simulink model "chap4_5sim"  (Simulink 7.7)
settings: Solver=ode45  StartTime=0.0  StopTime=10  RelTol=1e-5
settings Model: Creator=hp  LastModifiedBy=ljk  ExtModeTrigMode=oneshot  ExtModeArmWhenConnect=off
settings DataIOCC: LimitDataPoints=off  SignalLoggingName=sigsOut
settings OptimizationCC: BooleanDataType=off  InitFltsAndDblsToZero=on
settings DebuggingCC: SaveWithParameterizedLinksMsg=none  SignalResolutionControl=TryResolveAllWithWarning  SolverPrmCheckMsg=none  MultiTaskDSMMsg=warning  MultiTaskCondExecSysMsg=none  StrictBusMsg=None
settings HardwareCC: TargetUnknown=on
settings RTWCC: IncludeERTFirstTime=on
settings GRTTargetCC: TargetFcnLib=ansi_tfl_tmw.mat

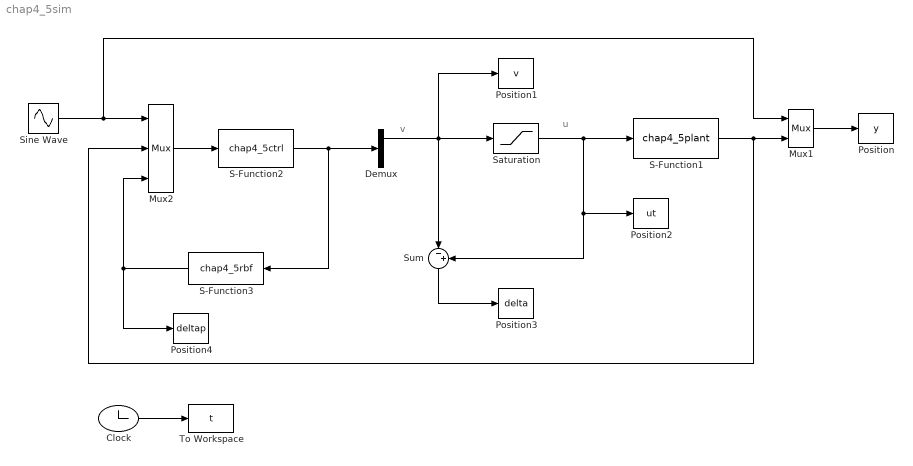
== system chap4_5sim ==
  note: v
  note: u
  Clock : Clock
      settings: Decimation=10
  Demux : Demux  Outputs=2
  Mux1 : Mux  Inputs=2
  Mux2 : Mux  Inputs=3
  Position : ToWorkspace  VariableName=y  SampleTime=-1  SaveFormat=Array
  Position1 : ToWorkspace  VariableName=v  SampleTime=-1  SaveFormat=Array
  Position2 : ToWorkspace  VariableName=ut  SampleTime=-1  SaveFormat=Array
  Position3 : ToWorkspace  VariableName=delta  SampleTime=-1  SaveFormat=Array
  Position4 : ToWorkspace  VariableName=deltap  SampleTime=-1  SaveFormat=Array
  S-Function1 : S-Function  FunctionName=chap4_5plant  EnableBusSupport=off
  S-Function2 : S-Function  FunctionName=chap4_5ctrl  EnableBusSupport=off
  S-Function3 : S-Function  FunctionName=chap4_5rbf  EnableBusSupport=off
  Saturation : Saturate  UpperLimit=3  LowerLimit=-3
  Sine Wave : Sin  SampleTime=0
  Sum : Sum  Inputs=|-+
  To Workspace : ToWorkspace  VariableName=t  SampleTime=-1  SaveFormat=Array
  wires:
  Mux1/1 -> Position/1
  S-Function1/1 -> Mux2/2, Mux1/2
  Clock/1 -> To Workspace/1
  Sine Wave/1 -> Mux2/1, Mux1/1
  Saturation/1 -> S-Function1/1, Position2/1, Sum/2
  Mux2/1 -> S-Function2/1
  S-Function2/1 -> Demux/1, S-Function3/1
  S-Function3/1 -> Mux2/3, Position4/1
  Sum/1 -> Position3/1
  Demux/1 -> Position1/1, Saturation/1, Sum/1
